simulink model "LQR_HIL_sim"  (R2021a)
settings: Solver=VariableStepAuto  StartTime=0.0  StopTime=60  RelTol=1e-3
values from neighbouring files (symbols this model uses):
  A = [0 1 0 0 ... (first row only)    [HIL_LQR.m]
  B = [0;b2;0;b4]    [HIL_LQR.m]
  C1 = [1 0 0 0 ... (first row only)    [HIL_LQR.m]
  Kr3 = inv(Cn*inv(-(A-B*K3))*B)    [HIL_LQR.m]
undefined symbols (not defined in the file or in its folder): LF
libraries: instrumentseriallib x3, svdutilitieslib x1
settings Model: Creator=Asus  LastModifiedBy=Asus

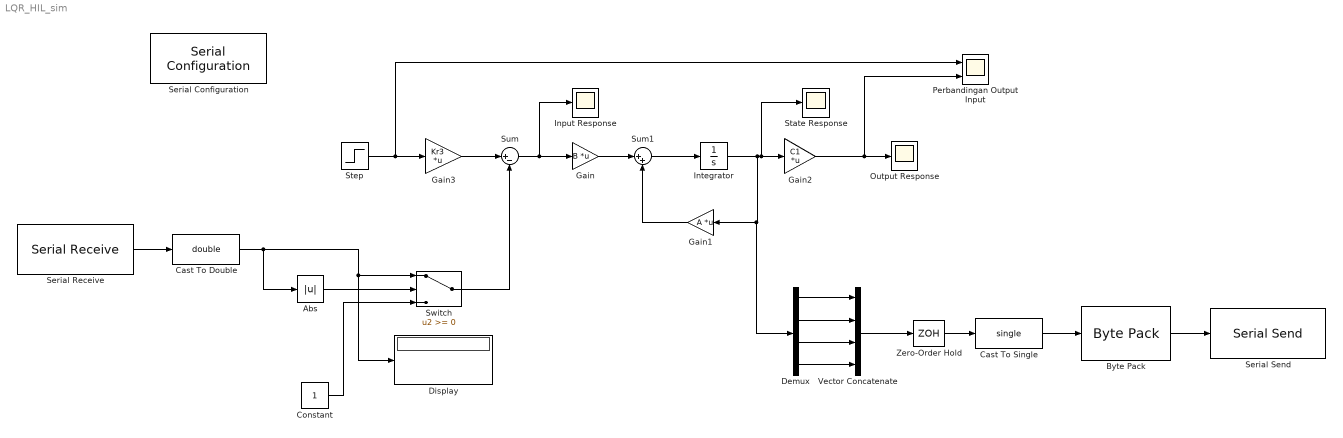
== system LQR_HIL_sim ==
  Abs : Abs
  Byte Pack : svdutilitieslib/Byte Pack  maskPackedDataType=uint8  datatypes={'single'}  byteAlign=1  blockPlatform=arduinoert
      settings: SourceProductBaseCode=ANDROID,ARDUINO,ML_ARDUINO,ECCORTEXA,ECCORTEXR,SC_BEAGLEBONE_BLUE,EC_FREEDOM_BOARD,EC_FRDM_K64F,INTEL_BLOCKSET,JETSONCPU,MICROBIT,NUCLEO,NVIDIA,PX4AUTOPILOTS,RASPPIIO,STMICRODIS,TIC2000,XILINX_BLOCKSET
  Cast To Double : DataTypeConversion  OutDataTypeStr=double
  Cast To Single : DataTypeConversion  OutDataTypeStr=single
  Constant : Constant
  Demux : Demux
  Display : Display
  Gain : Gain  Gain=B  Multiplication=Matrix(K*u)
  Gain1 : Gain  Gain=A  Multiplication=Matrix(K*u)
  Gain2 : Gain  Gain=C1  Multiplication=Matrix(K*u)
  Gain3 : Gain  Gain=Kr3  Multiplication=Matrix(K*u)
  Input Response : Scope
  Integrator : Integrator  InitialCondition=[0;0;0;0]
  Output Response : Scope
  Perbandingan Output Input : Scope  NumInputPorts=2
  Serial Configuration : instrumentseriallib/Serial Configuration  Priority=-200000  Port=COM36  ComPort=COM36  BaudRate=115200  DataBits=8  Parity=none  StopBits=1  ByteOrder=little-endian  FlowControl=none  Timeout=10  SimulateUsing=Interpreted execution  BlockInModel=on
  Serial Receive : instrumentseriallib/Serial Receive  Priority=1  Port=COM36  ComPort=COM36  DataType=single  SaveDataType=uint8  ToggleHeader=on  Header=[65]  ToggleTerminator=on  Terminator=LF ('\n')  CustomTerminator=[]  ToggleDataSize=on  DataSize=[1 1]  EnableBlockingMode=on  ActionDataUnavailable=Output custom value  ActionWhenDataUnavailable=Output custom value  CustomValue=0  SampleTime=0.05  SimulateUsing=Interpreted execution  BlockInModel=on
  Serial Send : instrumentseriallib/Serial Send  Priority=1  Port=COM36  ComPort=COM36  Header=['A']  Terminator=LF ('\n')  CustomTerminator=[]  EnableBlockingMode=on  SimulateUsing=Interpreted execution  BlockInModel=on
  State Response : Scope
  Step : Step  Time=0.5  SampleTime=0
  Sum : Sum  Inputs=|+-
  Sum1 : Sum  Inputs=|++
  Switch : Switch  ZeroCross=off
  Vector Concatenate : Concatenate  NumInputs=4
  Zero-Order Hold : ZeroOrderHold  SampleTime=0.05
  wires:
  Sum/1 -> Input Response/1, Gain/1
  Gain/1 -> Sum1/1
  Sum1/1 -> Integrator/1
  Gain1/1 -> Sum1/2
  Gain2/1 -> Perbandingan Output Input/2, Output Response/1
  Zero-Order Hold/1 -> Cast To Single/1
  Cast To Single/1 -> Byte Pack/1
  Byte Pack/1 -> Serial Send/1
  Serial Receive/1 -> Cast To Double/1
  Cast To Double/1 -> Abs/1, Display/1, Switch/1
  Gain3/1 -> Sum/1
  Step/1 -> Perbandingan Output Input/1, Gain3/1
  Integrator/1 -> State Response/1, Gain2/1, Demux/1, Gain1/1
  Demux/1 -> Vector Concatenate/1
  Demux/2 -> Vector Concatenate/2
  Demux/3 -> Vector Concatenate/3
  Demux/4 -> Vector Concatenate/4
  Vector Concatenate/1 -> Zero-Order Hold/1
  Constant/1 -> Switch/3
  Abs/1 -> Switch/2
  Switch/1 -> Sum/2
